simulink model "synchronous_motor_generator4"  (R2022b)
settings: Solver=VariableStepAuto  StartTime=0.0  StopTime=10.0  RelTol=1e-3
libraries: spsSynchronousMachineSIFundamentalLib x1, spsThreePhaseSeriesRLCLoadLib x1, spsThreePhaseSourceLib x1, spspowerguiLib x1
settings Model: Creator=Hessam  LastModifiedBy=Hessam

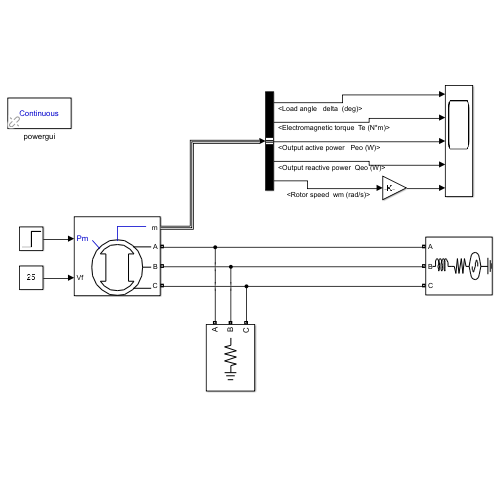
[thumbnail: Simulink's stored preview of the top-level diagram]
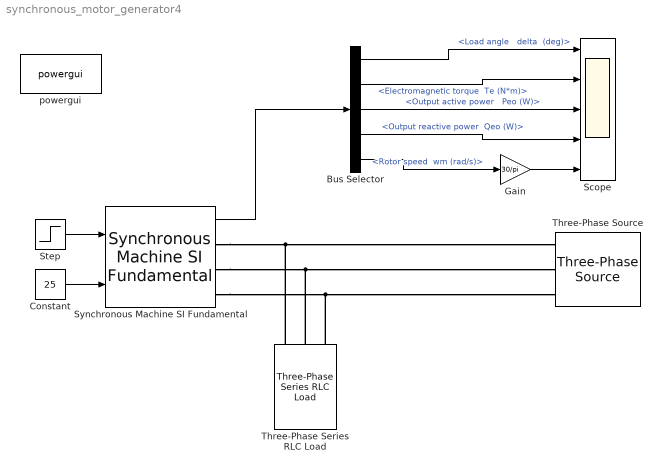
== system synchronous_motor_generator4 ==
  Bus Selector : BusSelector  OutputSignals="Load angle   delta  (deg),Mechanical.Electromagnetic torque  Te (N*m),Output active power   Peo (W),Output reactive power  Qeo (W),Mechanical.Rotor speed  wm (rad/s)"
  Constant : Constant  Value=25
  Gain : Gain  Gain=30/pi
  Scope : Scope  NumInputPorts=5
  Step : Step  Time=4  Before=-48864  After=60000  SampleTime=0
  Synchronous Machine SI Fundamental : spsSynchronousMachineSIFundamentalLib/Synchronous Machine SI Fundamental  PresetModel=No  MechanicalLoad=Mechanical power Pm  ShowDetailedParameters=on  RotorType=Salient-pole  Units=SI fundamental parameters  MeasurementBus=off  NominalParameters="[ 111.9E3  762.1024   60   0 ]"  Stator="[ 0.26  1.14E-3  13.7E-3  11E-3 ]"  Field="[ 0.13  2.1E-3 ]"  Dampers2=[ 0.0664, 1.387e-3, 0.0292, 6.896e-4, 7.907e-3, 2.477e-3]  Dampers1="[ 0.0224  1.4E-3  0.02  1E-3 ]"  Mechanical=[ 24.9 0 2 ]  PolePairs=20  InitialConditions="[ 0  -111.485  53.977  53.977  53.977  -173.297  -293.297  -53.2967  17.8876 ]"  SetSaturation=off  Saturation=[695.64,774.7,917.5,1001.6,1082.2,1175.9,1293.6,1430.2,1583.7;9660,10623,12243,13063,13757,14437,15180,15890,16567]  DisplayVfd=off  LoadFlowParameters=[1,0,0,0,0]  TsPowergui=0  TsBlock=-1  IterativeModel=Trapezoidal non iterative  IterativeDiscreteModel=Trapezoidal non iterative  BusType=PV  Pref=-50000  Qref=0  Qmin=-inf  Qmax=inf  PLF=0  QLF=0
      settings: LibrarySourceBlock=|
      | sps_lib/Electrical Machines/Synchronous Machine
      | SI Fundamental
  Three-Phase Series RLC Load : spsThreePhaseSeriesRLCLoadLib/Three-Phase Series RLC Load  LConnTagsString=A|B|C  Configuration=Y (grounded)  NominalVoltage=762  Vabc=[1e3 1e3 1e3]  Vabcp=[1e3 1e3 1e3]  NominalFrequency=60  UnbalancedPower=off  ActivePower=11e3  InductivePower=0  CapacitivePower=0  Pabc=[10e3 9e3 11e3]  QLabc=[100 90 110]  QCabc=[100 90 110]  Pabcp=[10e3 9e3 11e3]  QLabcp=[100 90 110]  QCabcp=[100 90 110]  Measurements=None  LoadType=constant Z
  Three-Phase Source : spsThreePhaseSourceLib/Three-Phase Source  InternalConnection=Yg  VoltagePhases=off  Voltage=762.1  PhaseAngle=0  Voltage_phases=[25e3 25e3 25e3]/sqrt(3)  PhaseAngles_phases=[0 -120 +120]  Frequency=60  NonIdealSource=on  SpecifyImpedance=off  Resistance=762^2/10e6/10  Inductance=762^2/10e6/(2*pi*60)  ShortCircuitLevel=100e6  BaseVoltage=25e3  XRratio=7  BusType=swing  Pref=10e3  Qref=0  Prefabc=[10e3, 10e3, 10e3]  Qrefabc=[0, 0, 0]  Qmin=-inf  Qmax=inf
  powergui : spspowerguiLib/powergui  Priority=1  SimulationMode=Continuous  SampleTime=50e-6  frequency=60  Iterations=50  frequencyindice=60  Pbase=100e6  ErrMax=1e-4  UnitsV=kV  UnitsW=MW  buscounter=0  FunctionMessages=off  echomessages=off  EnableUseOfTLC=off  CurrentSourceSwitches=off  DisableSnubberDevices=off  DisableRonSwitches=off  DisableVfSwitches=off  DisplayEquations=off  AutomaticDiscreteSolvers=off  SolverType=Tustin/Backward Euler (TBE)  Interpol=off  ExternalGateDelay=off  methode=off  Ts=100  x0status=blocks  SPID=on  SwTol=0  HookPort=off  NonlinearTolerance=1e-4  nMaxIteration=100  ContinueOnMaxIteration=off  RestoreLinks=warning  ResistiveCurrentMeasurement=off  Frange=[0:2:500]  Ylog=off  Xlog=on  ShowGrid=off  save=off  variable=ZData  structure=0  ZoomFFT=off  StartTime=0.0  cycles=1  DisplayStyle=1  fundamental=60  FreqAxis=off  MaxFrequency=1000  frequencyindicesteady=1  RmsSteady=1  display=off
  wires:
  Step/1 -> Synchronous Machine SI Fundamental/1
  Constant/1 -> Synchronous Machine SI Fundamental/2
  Synchronous Machine SI Fundamental/1 -> Bus Selector/1
  Bus Selector/3 -> Scope/3  "<Output active power   Peo (W)>"
  Bus Selector/2 -> Scope/2  "<Electromagnetic torque  Te (N*m)>"
  Bus Selector/1 -> Scope/1  "<Load angle   delta  (deg)>"
  Bus Selector/4 -> Scope/4  "<Output reactive power  Qeo (W)>"
  Bus Selector/5 -> Gain/1  "<Rotor speed  wm (rad/s)>"
  Gain/1 -> Scope/5
  connections:
  Synchronous Machine SI Fundamental/RConn1 -- Three-Phase Series RLC Load/LConn1 -- Three-Phase Source/RConn1
  Synchronous Machine SI Fundamental/RConn2 -- Three-Phase Series RLC Load/LConn2 -- Three-Phase Source/RConn2
  Synchronous Machine SI Fundamental/RConn3 -- Three-Phase Series RLC Load/LConn3 -- Three-Phase Source/RConn3
